simulink model "FPGA_Prova1_fixedpoint"  (R2023b)
settings: Solver=VariableStepAuto  StartTime=0.0  StopTime=10.0  RelTol=1e-3
libraries: hwlogicconnlib x2
settings Model: Creator=lenovo GAME  LastModifiedBy=lenovo GAME

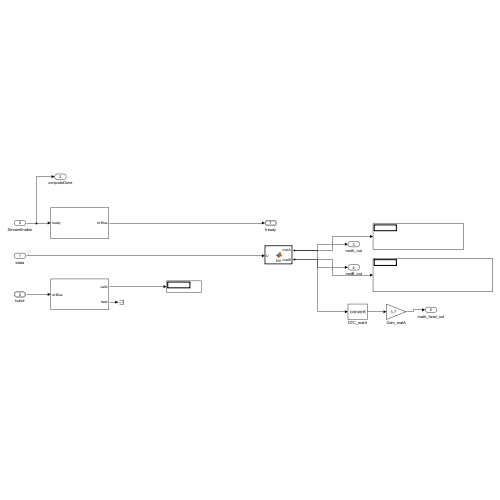
[thumbnail: Simulink's stored preview of the top-level diagram]
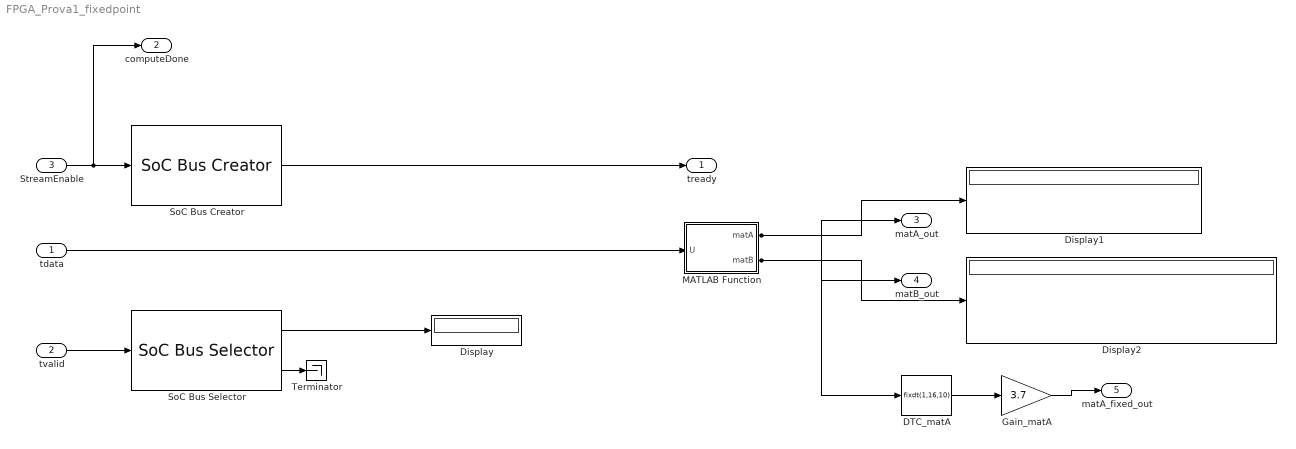
== system FPGA_Prova1_fixedpoint ==
  tdata : Inport  OutDataTypeStr=fixdt(1,32,16)  PortDimensions=25  SampleTime=1e-08
  tvalid : Inport  Port=2  OutDataTypeStr=Bus: StreamM2SBusObj  SampleTime=1e-08
  StreamEnable : Inport  Port=3  SampleTime=1e-08
  DTC_matA : DataTypeConversion  OutDataTypeStr=fixdt(1,16,10)  SaturateOnIntegerOverflow=off  RndMeth=Floor
  Display : Display
  Display1 : Display
  Display2 : Display
  Gain_matA : Gain  Gain=3.7  OutDataTypeStr=fixdt(1,16,10)
  MATLAB Function : MATLAB Function  TreatAsAtomicUnit=on
  SoC Bus Creator : hwlogicconnlib/SoC Bus Creator  Protocol=Data stream  ctrltype=Ready
  SoC Bus Selector : hwlogicconnlib/SoC Bus Selector  Protocol=Data stream  ctrltype=Valid
  Terminator : Terminator
  tready : Outport  OutDataTypeStr=Bus: StreamS2MBusObj
  computeDone : Outport  Port=2
  matA_out : Outport  Port=3
  matB_out : Outport  Port=4
  matA_fixed_out : Outport  Port=5
  wires:
  tvalid/1 -> SoC Bus Selector/1
  SoC Bus Selector/2 -> Terminator/1
  SoC Bus Selector/1 -> Display/1
  StreamEnable/1 -> SoC Bus Creator/1, computeDone/1
  SoC Bus Creator/1 -> tready/1
  tdata/1 -> MATLAB Function/1(U)
  MATLAB Function/2(matB) -> Display2/1, matB_out/1
  MATLAB Function/1(matA) -> Display1/1, matA_out/1, DTC_matA/1
  DTC_matA/1 -> Gain_matA/1
  Gain_matA/1 -> matA_fixed_out/1

== matlab function FPGA_Prova1_fixedpoint/MATLAB Function ==
  data: U input; matA output; matB output
function [matA, matB] = fcn(U)   % U è 25x1 double
matA = reshape(U(1:9), [3 3]);
matB = reshape(U(10:25), [4 4]);
end
